simulink model "LQR_method"  (R2018b)
settings: Solver=FixedStepDiscrete  StartTime=0.0  StopTime=inf  FixedStep=TS  RelTol=1e-3  EnableMultiTasking=on
values from neighbouring files (symbols this model uses):
  ES = -C2DEG*D2R    (= -0.00872664625997)    [parameter.m]
  GS = GyroS*D2R    [parameter.m]
  KLQR = [-500,-25,5,47]    [parameter.m]
  r_w = 0.016    [final.m]    (also in parameter.m)
  TS = 0.005    [parameter.m]
  tstart = .6    (= 0.6)    [parameter.m]
  V2DCB = 1/DCB2V    (= 28.3333333333)    [parameter.m]
libraries: simulink x2, arduinolib x2, MinSegLibrary_M1V4 x1
settings Model: SimulationMode=external  ExtModeTrigDuration=2  Creator=luyey  LastModifiedBy=luyey
settings OptimizationCC: EnhancedBackFolding=on  PassReuseOutputArgsAs=Individual arguments  MaxStackSize=64  OptimizeBlockOrder=speed  DifferentSizesBufferReuse=on  OptimizationCustomize=off
settings DebuggingCC: ParameterTunabilityLossMsg=error
settings HardwareCC: ProdBitPerInt=16  ProdBitPerPointer=16  ProdBitPerSizeT=16  ProdBitPerPtrDiffT=16  ProdLargestAtomicFloat=None  ProdWordSize=8  ProdHWDeviceType=Atmel->AVR  UseEmbeddedCoderFeatures=off  UseSimulinkCoderFeatures=off
settings ModelReferenceCC: PropagateSignalLabelsOutOfModel=off
settings SFSimCC: MATLABDynamicMemAlloc=off
settings RTWCC: SystemTargetFile=ert.tlc  HardwareBoard=Arduino Mega 2560  TemplateMakefile=ert_default_tmf  GenerateReport=on  Toolchain=Arduino AVR  BuildConfiguration=Faster Runs  IncludeHyperlinkInReport=on  LaunchReport=on  GenerateTraceInfo=on  GenerateTraceReport=on  GenerateTraceReportSl=on  GenerateTraceReportSf=on  GenerateTraceReportEml=on
settings CodeAppCC: ForceParamTrailComments=on  IgnoreCustomStorageClasses=off  OperatorAnnotations=on  SimulinkDataObjDesc=on  SFDataObjDesc=on  MangleLength=10  InsertBlockDesc=on
settings ERTTargetCC: SupportContinuousTime=on  SupportNonInlinedSFcns=on  SupportVariableSizeSignals=on

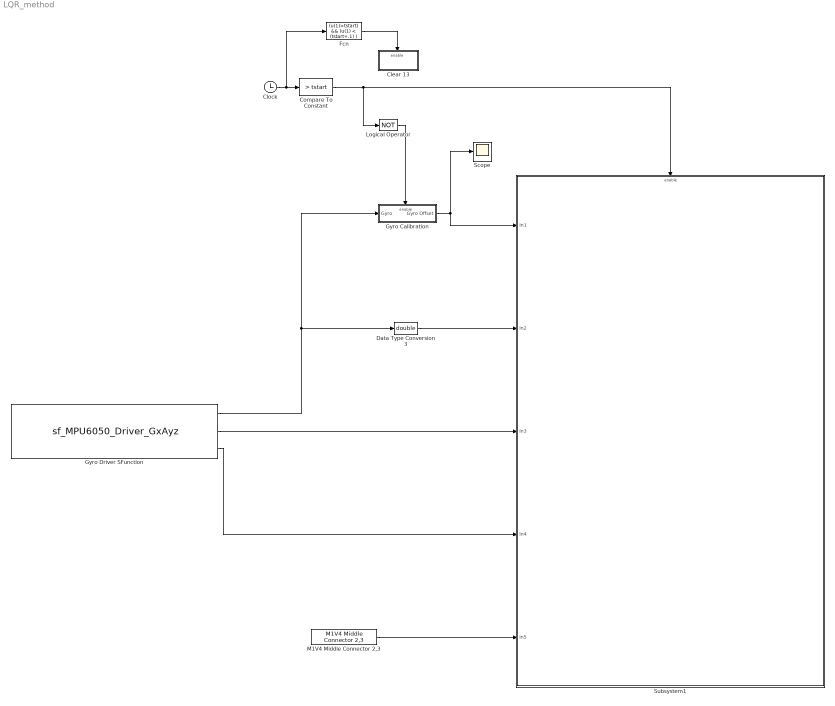
== system LQR_method ==
  "Clear 13 " : Subsystem  TreatAsAtomicUnit=on
  Clock : Clock
  Compare To Constant : simulink/Logic and Bit Operations/Compare To Constant  relop=>  const=tstart  OutDataTypeStr=boolean
  Data Type Conversion3 : DataTypeConversion  OutDataTypeStr=double
  Fcn : Fcn  Expr=(u(1)>tstart) && (u(1) < (tstart+.1) )
  Gyro Calibration : Subsystem  TreatAsAtomicUnit=on
  Gyro Driver SFunction : S-Function  InitFcn=try, set_param(gcb,'FunctionName','sf_MPU6050_Driver_GxAyz'), end  FunctionName=sf_MPU6050_Driver_GxAyz  SFunctionModules=sf_MPU6050_Driver_GxAyz_wrapper  SFunctionDeploymentMode=off  EnableBusSupport=off  mask(S-Function Builder){}
      mask help: Simulink:masks:SFunctionBuilder_MD
      mask init:
      | val = [[.9  0.75 0.75 1 1 .9 .9 1]',[1 1 0.75 0.75 .9 .9 1 .9]'];try , sys = get_param(gcb,'SfunBuilderFcnName');if isempty(sys), sys = get_param(gcb,'FunctionName'); end,catch, sys = get_param(gcb,'FunctionName'); end
      settings: CopyFcn=set_param(gcbh,'LinkStatus','none')  PreSaveFcn=try, set_param(gcb,'FunctionName','sf_MPU6050_Driver_GxAyz'), end  OpenFcn=sfunctionwizard(gcbh)
      mask Display: plot(val(:,1),val(:,2)),disp(sys), port_label('output',1,'x_vel'), port_label('output',2,'y_acc'), port_label('output',3,'z_acc')
  Logical Operator : Logic  Operator=NOT  AllPortsSameDT=off  OutDataTypeStr=boolean
  M1V4 Middle Connector 2,3 : MinSegLibrary_M1V4/M1V4 Middle Connector 2,3  Encoder=3  PinA=15  PinB=62
      settings: SourceProductName=Rensselaer Arduino Support Package
  Scope : Scope
  Subsystem1 : Subsystem
  wires:
  Data Type Conversion3/1 -> Subsystem1/2(In2)
  Gyro Driver SFunction/2 -> Subsystem1/3(In3)
  Gyro Driver SFunction/3 -> Subsystem1/4(In4)
  M1V4 Middle Connector 2,3/1 -> Subsystem1/5(In5)
  Gyro Driver SFunction/1 -> Gyro Calibration/1(Gyro), Data Type Conversion3/1
  Compare To Constant/1 -> Subsystem1/Enable, Logical Operator/1
  Gyro Calibration/1(Gyro Offset) -> Subsystem1/1(In1), Scope/1
  Clock/1 -> Fcn/1, Compare To Constant/1
  Logical Operator/1 -> Gyro Calibration/Enable
  Fcn/1 -> "Clear 13 "/Enable

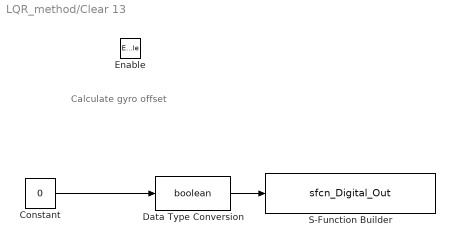
== system LQR_method/Clear 13  ==
  note: Calculate gyro offset
  Enable : EnablePort
  Constant : Constant  Value=0
  Data Type Conversion : DataTypeConversion  OutDataTypeStr=boolean
  S-Function Builder : S-Function  InitFcn=try, set_param(gcb,'FunctionName','sfcn_Digital_Out'), end  FunctionName=sfcn_Digital_Out  Parameters=uint8(13)  SFunctionModules=sfcn_Digital_Out_wrapper  SFunctionDeploymentMode=off  EnableBusSupport=off  mask(S-Function Builder){}
      mask init: same as LQR_method/Gyro Driver SFunction
      settings: CopyFcn=set_param(gcbh,'LinkStatus','none')  PreSaveFcn=try, set_param(gcb,'FunctionName','sfcn_Digital_Out'), end  OpenFcn=sfunctionwizard(gcbh)
      mask Display: plot(val(:,1),val(:,2)),disp(sys), port_label('input',1,'in')
  wires:
  Data Type Conversion/1 -> S-Function Builder/1
  Constant/1 -> Data Type Conversion/1

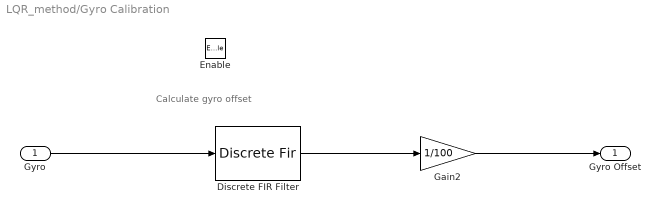
== system LQR_method/Gyro Calibration ==
  note: Calculate gyro offset
  Gyro : Inport
  Enable : EnablePort
  Discrete FIR Filter : DiscreteFir  Coefficients=ones(1,100)
  Gain2 : Gain  Gain=1/100  OutDataTypeStr=Inherit: Same as input  ParamDataTypeStr=Inherit: Same as input
  Gyro Offset : Outport
  wires:
  Gyro/1 -> Discrete FIR Filter/1
  Discrete FIR Filter/1 -> Gain2/1
  Gain2/1 -> Gyro Offset/1

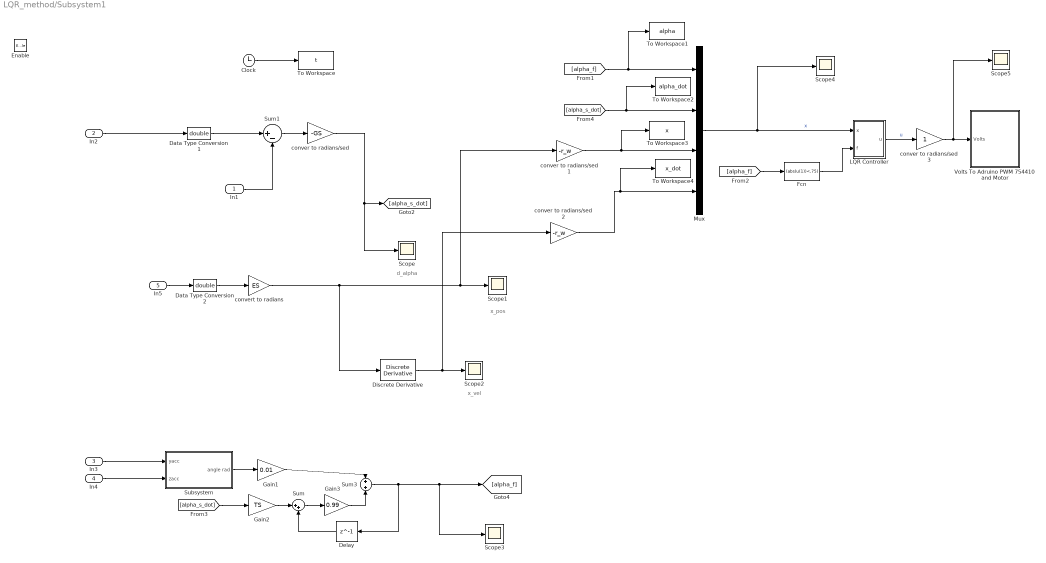
== system LQR_method/Subsystem1 ==
  note: d_alpha
  note: x_pos
  note: x_vel
  In1 : Inport
  In2 : Inport  Port=2
  In3 : Inport  Port=3
  In4 : Inport  Port=4
  In5 : Inport  Port=5
  Enable : EnablePort
  Clock : Clock
  Data Type Conversion1 : DataTypeConversion  OutDataTypeStr=double
  Data Type Conversion2 : DataTypeConversion  OutDataTypeStr=double
  Delay : Delay  DelayLength=1  InitialCondition=0
  Discrete Derivative : simulink/Discrete/Discrete Derivative  gainval=1.0  ICPrevScaledInput=0.0  OutMin=[]  OutMax=[]  OutDataType=fixdt(1, 16)  OutScaling=2^-10  DoSatur=off
  Fcn : Fcn  Expr=(abs(u(1))<.75)
  Gain1 : Gain  Gain=0.01
  Gain2 : Gain  Gain=TS
  Gain3 : Gain  Gain=0.99
  LQR Controller : Subsystem
  Mux : Mux
  Scope{,1..5} (6 alike) : Scope
  Subsystem : Subsystem
  Sum : Sum  Inputs=|++
  Sum1 : Sum  Inputs=|+-
  Sum3 : Sum
  To Workspace : ToWorkspace  VariableName=t  SaveFormat=Timeseries  SampleTime=-1
  To Workspace1 : ToWorkspace  VariableName=alpha  SampleTime=-1
  To Workspace2 : ToWorkspace  VariableName=alpha_dot  SampleTime=-1
  To Workspace3 : ToWorkspace  VariableName=x  SampleTime=-1
  To Workspace4 : ToWorkspace  VariableName=x_dot  SampleTime=-1
  Volts To Adruino PWM 754410 and Motor : Subsystem
  conver to radians/sed : Gain  Gain=-GS
  conver to radians/sed1 : Gain  Gain=-r_w
  conver to radians/sed2 : Gain  Gain=-r_w
  conver to radians/sed3 : Gain
  convert to radians : Gain  Gain=ES  OutDataTypeStr=double
  wires:
  Gain3/1 -> Sum3/2
  conver to radians/sed/1 -> [alpha_s_dot], Scope/1
  Gain2/1 -> Sum/1
  convert to radians/1 -> Discrete Derivative/1, conver to radians/sed1/1, Scope1/1
  In2/1 -> Data Type Conversion1/1
  In4/1 -> Subsystem/2(zacc)
  In3/1 -> Subsystem/1(yacc)
  Data Type Conversion2/1 -> convert to radians/1
  Sum3/1 -> Scope3/1, [alpha_f], Delay/1
  Fcn/1 -> LQR Controller/2(f)
  In1/1 -> Sum1/2
  Discrete Derivative/1 -> conver to radians/sed2/1, Scope2/1
  [alpha_f] -> Fcn/1
  Data Type Conversion1/1 -> Sum1/1
  Delay/1 -> Sum/2
  Sum1/1 -> conver to radians/sed/1
  In5/1 -> Data Type Conversion2/1
  conver to radians/sed2/1 -> To Workspace4/1, Mux/4
  Sum/1 -> Gain3/1
  Gain1/1 -> Sum3/1
  Subsystem/1(angle rad) -> Gain1/1
  [alpha_s_dot] -> Gain2/1
  Mux/1 -> Scope4/1, LQR Controller/1(x)  "x"
  conver to radians/sed1/1 -> To Workspace3/1, Mux/3
  [alpha_f] -> To Workspace1/1, Mux/1
  [alpha_s_dot] -> To Workspace2/1, Mux/2
  conver to radians/sed3/1 -> Scope5/1, Volts To Adruino PWM 754410 and Motor/1(Volts)
  LQR Controller/1(u) -> conver to radians/sed3/1  "u"
  Clock/1 -> To Workspace/1

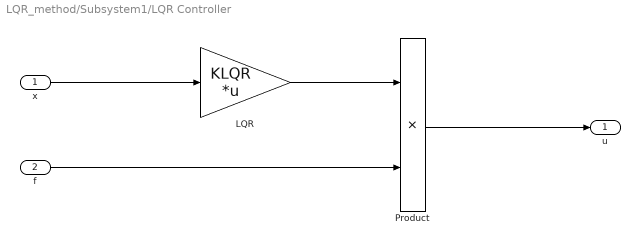
== system LQR_method/Subsystem1/LQR Controller ==
  x : Inport
  f : Inport  Port=2
  LQR : Gain  Gain=KLQR  Multiplication=Matrix(K*u)
  Product : Product  RndMeth=Zero
  u : Outport
  wires:
  x/1 -> LQR/1
  LQR/1 -> Product/1
  Product/1 -> u/1
  f/1 -> Product/2

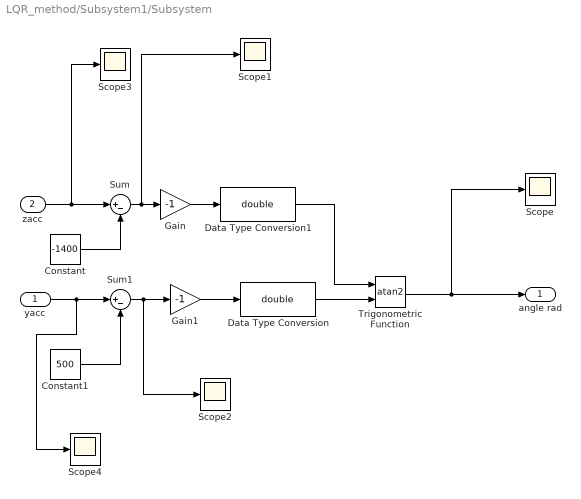
== system LQR_method/Subsystem1/Subsystem ==
  yacc : Inport
  zacc : Inport  Port=2
  Constant : Constant  Value=-1400
  Constant1 : Constant  Value=500
  Data Type Conversion : DataTypeConversion  OutDataTypeStr=double
  Data Type Conversion1 : DataTypeConversion  OutDataTypeStr=double
  Gain : Gain  Gain=-1
  Gain1 : Gain  Gain=-1
  Scope{,1..4} (5 alike) : Scope
  Sum : Sum  Inputs=|+-
  Sum1 : Sum  Inputs=|+-
  Trigonometric Function : Trigonometry  Operator=atan2
  angle rad : Outport
  wires:
  Trigonometric Function/1 -> Scope/1, angle rad/1
  Data Type Conversion1/1 -> Trigonometric Function/1
  Data Type Conversion/1 -> Trigonometric Function/2
  zacc/1 -> Scope3/1, Sum/1
  yacc/1 -> Scope4/1, Sum1/1
  Constant/1 -> Sum/2
  Constant1/1 -> Sum1/2
  Sum/1 -> Scope1/1, Gain/1
  Gain/1 -> Data Type Conversion1/1
  Sum1/1 -> Scope2/1, Gain1/1
  Gain1/1 -> Data Type Conversion/1

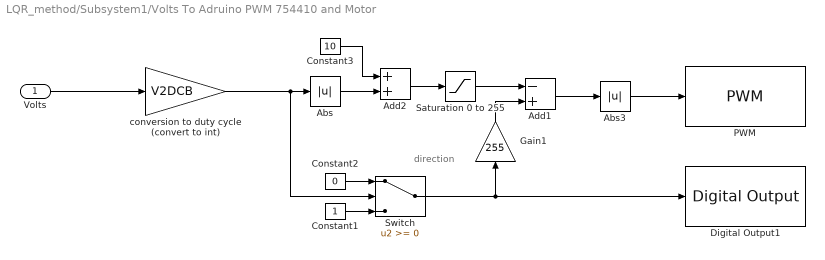
== system LQR_method/Subsystem1/Volts To Adruino PWM 754410 and Motor ==
  note: direction
  Volts : Inport
  Abs : Abs
  Abs3 : Abs
  Add1 : Sum  Inputs=-+
  Add2 : Sum
  Constant1 : Constant
  Constant2 : Constant  Value=0
  Constant3 : Constant  Value=10
  Digital Output1 : arduinolib/Digital Output  pinNumber=2  blockPlatform=arduino
  Gain1 : Gain  Gain=255
  PWM : arduinolib/PWM  pinNumber=5  EnableInputFrequency=off  InitialFrequency=2000  InitialDutyCycle=0  NotificationType=None  blockPlatform=arduino
  Saturation 0 to 255 : Saturate  UpperLimit=255  LowerLimit=0
  Switch : Switch
  conversion to duty cycle (convert to int) : Gain  Gain=V2DCB  OutDataTypeStr=int16
  wires:
  Constant3/1 -> Add2/1
  Abs/1 -> Add2/2
  Abs3/1 -> PWM/1
  Add2/1 -> Saturation 0 to 255/1
  Add1/1 -> Abs3/1
  conversion to duty cycle (convert to int)/1 -> Switch/2, Abs/1
  Volts/1 -> conversion to duty cycle (convert to int)/1
  Constant2/1 -> Switch/1
  Switch/1 -> Digital Output1/1, Gain1/1
  Gain1/1 -> Add1/2
  Saturation 0 to 255/1 -> Add1/1
  Constant1/1 -> Switch/3
